simulink model "Cv_12"  (R2024a)
settings: Solver=VariableStepAuto  StartTime=0.0  StopTime=10.0  RelTol=1e-3
undefined symbols (not defined in the file): b, J, K, L, R
settings Model: Creator=Miloš Uhlíř  LastModifiedBy=Miloš Uhlíř

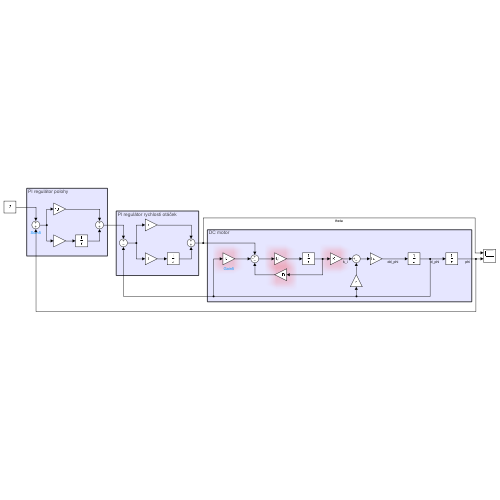
[thumbnail: Simulink's stored preview of the top-level diagram]
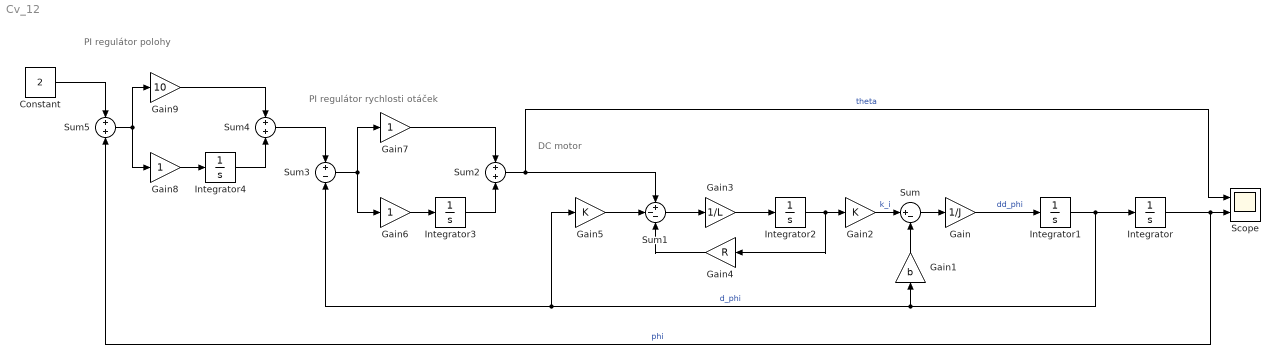
== system Cv_12 ==
  note: PI regulátor polohy
  note: PI regulátor rychlosti otáček
  note: DC motor
  Constant : Constant  Value=2
  Gain : Gain  Gain=1/J
  Gain1 : Gain  Gain=b
  Gain2 : Gain  Gain=K
  Gain3 : Gain  Gain=1/L
  Gain4 : Gain  Gain=R
  Gain5 : Gain  Gain=K
  Gain6 : Gain
  Gain7 : Gain
  Gain8 : Gain
  Gain9 : Gain  Gain=10
  Integrator{,1..4} (5 alike) : Integrator
  Scope : Scope  NumInputPorts=2
  Sum : Sum  Inputs=|+-
  Sum1 : Sum  Inputs=+--
  Sum2 : Sum
  Sum3 : Sum  Inputs=+-
  Sum4 : Sum
  Sum5 : Sum
  wires:
  Integrator/1 -> Sum5/2, Scope/2  "phi"
  Integrator1/1 -> Sum3/2, Gain5/1, Gain1/1, Integrator/1  "d_phi"
  Gain/1 -> Integrator1/1  "dd_phi"
  Sum/1 -> Gain/1
  Gain2/1 -> Sum/1  "k_i"
  Gain1/1 -> Sum/2
  Gain3/1 -> Integrator2/1
  Integrator2/1 -> Gain4/1, Gain2/1
  Sum1/1 -> Gain3/1
  Gain4/1 -> Sum1/3
  Gain5/1 -> Sum1/2
  Sum2/1 -> Sum1/1, Scope/1  "theta"
  Gain6/1 -> Integrator3/1
  Integrator3/1 -> Sum2/2
  Gain7/1 -> Sum2/1
  Sum3/1 -> Gain7/1, Gain6/1
  Integrator4/1 -> Sum4/2
  Gain9/1 -> Sum4/1
  Gain8/1 -> Integrator4/1
  Sum4/1 -> Sum3/1
  Sum5/1 -> Gain8/1, Gain9/1
  Constant/1 -> Sum5/1
